simulink model "Loadcell"  (R2024b)
settings: Solver=FixedStepAuto  StartTime=0.0  StopTime=1  FixedStep=0.01  RelTol=1e-3  EnableMultiTasking=on
libraries: stm32f4xxblockslib x1
settings Model: STM32="{\"AnalogInput\":[{\"ID\":\"untitled:4\"},{\"ID\":\"Loadcell:4\"}]}"  Creator=admin  LastModifiedBy=admin
settings OptimizationCC: DefaultParameterBehavior=Inlined  EnhancedBackFolding=on  PassReuseOutputArgsAs=Individual arguments  ZeroExternalMemoryAtStartup=off  ZeroInternalMemoryAtStartup=off  MaxStackSize=512  OptimizeBlockOrder=speed  DifferentSizesBufferReuse=on  OptimizationCustomize=off  EfficientTunableParamExpr=on
settings DebuggingCC: ParameterTunabilityLossMsg=error
settings HardwareCC: ProdBitPerPointer=32  ProdBitPerSizeT=32  ProdBitPerPtrDiffT=32  ProdLargestAtomicInteger=Long  ProdLargestAtomicFloat=Double  ProdWordSize=32  ProdLongLongMode=on  ProdHWDeviceType=ARM Compatible->ARM Cortex-M
settings SFSimCC: MATLABDynamicMemAlloc=off
settings RTWCC: Description=Embedded Coder  SystemTargetFile=ert.tlc  HardwareBoard=STM32G4xx Based  TemplateMakefile=ert_default_tmf  Toolchain=GNU Tools for ARM Embedded Processors
settings CodeAppCC: ForceParamTrailComments=on  IgnoreCustomStorageClasses=off  OperatorAnnotations=on  SimulinkDataObjDesc=on  SFDataObjDesc=on  InsertBlockDesc=on
settings ERTTargetCC: TargetLangStandard=C99 (ISO)  CodeReplacementLibrary=ARM Cortex-M  ExtModeTransport=3  ExtModeStaticAlloc=on  ExtModeStaticAllocSize=2048  ExtModeMexFile=ext_xcp  ExtModeIntrfLevel=Level2 - Open

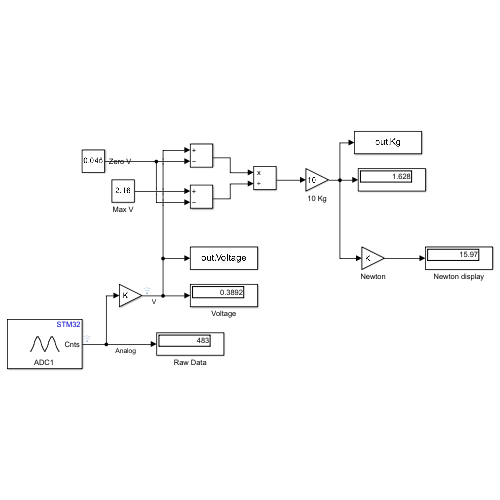
[thumbnail: Simulink's stored preview of the top-level diagram]
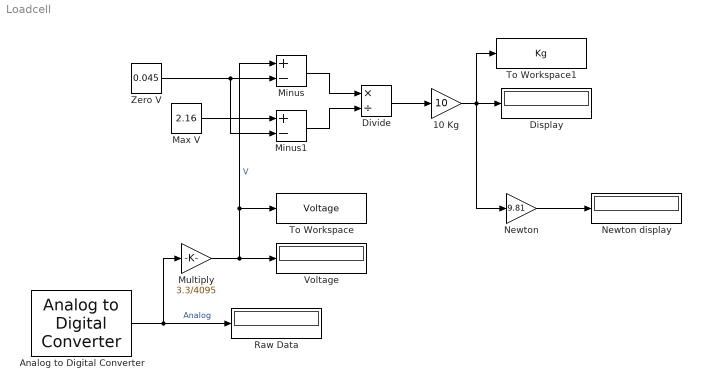
== system Loadcell ==
  10 Kg : Gain  Gain=10
  Analog to Digital Converter : stm32f4xxblockslib/Analog to Digital Converter  ADCModule=ADC1  ConversionGroup=Regular  TriggerMode=Trigger and read  NumberOfConversions=1  EnableBufferConv=off  BufferLength=1  OutputStatus=off  SampleTime=-1  EnableSimPort=off  hoistedMaskSrc=ECSoC/ECSimCodegen/Analog to Digital Converter
  Display : Display
  Divide : Product  Inputs=*/
  Max V : Constant  Value=2.16
  Minus : Sum  Inputs=+-
  Minus1 : Sum  Inputs=+-
  Multiply : Gain  Gain=3.3/4095
  Newton : Gain  Gain=9.81
  Newton display : Display
  Raw Data : Display
  To Workspace : ToWorkspace  VariableName=Voltage  SampleTime=-1
      settings: Save2DSignal=2-D array (concatenate along first dimension)
  To Workspace1 : ToWorkspace  VariableName=Kg  SampleTime=-1
      settings: Save2DSignal=2-D array (concatenate along first dimension)
  Voltage : Display
  Zero V : Constant  Value=0.045
  wires:
  Analog to Digital Converter/1 -> Multiply/1, Raw Data/1  "Analog"
  Multiply/1 -> To Workspace/1, Minus/1, Voltage/1  "V"
  Zero V/1 -> Minus1/2, Minus/2
  Max V/1 -> Minus1/1
  Minus/1 -> Divide/1
  Minus1/1 -> Divide/2
  Divide/1 -> 10 Kg/1
  10 Kg/1 -> Newton/1, Display/1, To Workspace1/1
  Newton/1 -> Newton display/1
